simulink model "Quad"  (R2015a)
settings: Solver=ode3  StartTime=0.0  StopTime=10  FixedStep=0.01  RelTol=1e-3
settings Model: Creator=Nick  LastModifiedBy=Nick

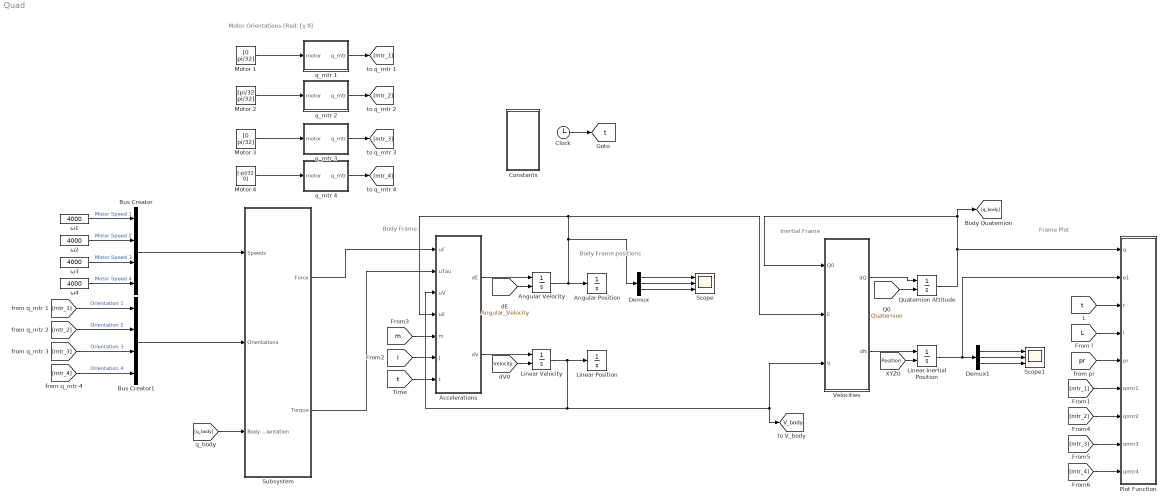
== system Quad ==
  note: Motor Orientations
      | (Rad: [γ δ]
  note: Frame Plot
  note: Inertial Frame
  note: Body Frame
      | positions
  note: Body Frame
  Accelerations : MATLAB Function  TreatAsAtomicUnit=on
  Angular Position : Integrator
  Angular Velocity : Integrator  InitialConditionSource=external
  Bus Creator : BusCreator
  Bus Creator1 : BusCreator
  Clock : Clock
  Constants : Subsystem
  Demux : Demux  Outputs=3
  Demux1 : Demux  Outputs=3
  Linear Inertial Position : Integrator  InitialConditionSource=external
  Linear Position : Integrator
  Linear Velocity : Integrator  InitialConditionSource=external
  Motor 1 : Constant  Value=[0 pi/32]
  Motor 2 : Constant  Value=[pi/32 pi/32]
  Motor 3 : Constant  Value=[0 pi/32]
  Motor 4 : Constant  Value=[-pi/32 0]
  Plot Function : MATLAB Function  TreatAsAtomicUnit=on
  Quaternion Attitude : Integrator  InitialConditionSource=external  ContinuousStateAttributes='Quaternion'
  Scope : Scope  NumInputPorts=3
      settings: YMin=-5~-5~-5  YMax=5~5~5
  Scope1 : Scope  NumInputPorts=3
      settings: YMin=-5~-5~-5  YMax=5~5~5
  Subsystem : Subsystem
  Velocities : MATLAB Function  TreatAsAtomicUnit=on
  q_mtr 1 : MATLAB Function  TreatAsAtomicUnit=on
  q_mtr 2 : MATLAB Function  TreatAsAtomicUnit=on
  q_mtr 3 : MATLAB Function  TreatAsAtomicUnit=on
  q_mtr 4 : MATLAB Function  TreatAsAtomicUnit=on
  ω{1..4} (4 alike) : Constant  Value=4000
  tag scope: V_body=global, t=global
  wires:
  [L] -> Plot Function/4(l)
  [pr] -> Plot Function/5(pr)
  Clock/1 -> [t]
  [t] -> Plot Function/3(t)
  [t] -> Accelerations/7(t)
  [I] -> Accelerations/6(J)
  [m] -> Accelerations/5(m)
  Accelerations/1(dE) -> Angular Velocity/1
  Angular Velocity/1 -> Demux/1, Accelerations/4(uE), Velocities/2(E), Angular Position/1
  Accelerations/2(dV) -> Linear Velocity/1
  Linear Velocity/1 -> Accelerations/3(uV), Velocities/3(V), [V_body], Linear Position/1
  Demux/1 -> Scope/1
  Demux/2 -> Scope/2
  Demux/3 -> Scope/3
  Demux1/1 -> Scope1/1
  Demux1/2 -> Scope1/2
  Demux1/3 -> Scope1/3
  [Velocity] -> Linear Velocity/2
  [Angular_Velocity] -> Angular Velocity/2
  Velocities/2(dN) -> Linear Inertial Position/1
  [Position] -> Linear Inertial Position/2
  Linear Inertial Position/1 -> Demux1/1, Plot Function/2(e1)
  [Quaternion] -> Quaternion Attitude/2
  Velocities/1(dQ) -> Quaternion Attitude/1
  Quaternion Attitude/1 -> [q_body], Velocities/1(Q0), Plot Function/1(q)
  Motor 1/1 -> q_mtr 1/1(motor)
  Motor 2/1 -> q_mtr 2/1(motor)
  Motor 3/1 -> q_mtr 3/1(motor)
  Motor 4/1 -> q_mtr 4/1(motor)
  q_mtr 1/1(q_mtr) -> [mtr_1]
  q_mtr 4/1(q_mtr) -> [mtr_4]
  q_mtr 3/1(q_mtr) -> [mtr_3]
  q_mtr 2/1(q_mtr) -> [mtr_2]
  [mtr_1] -> Plot Function/6(qmtr1)
  [mtr_2] -> Plot Function/7(qmtr2)
  [mtr_3] -> Plot Function/8(qmtr3)
  [mtr_4] -> Plot Function/9(qmtr4)
  [q_body] -> Subsystem/3(Body Orientation)
  Subsystem/1(Force) -> Accelerations/1(uF)
  Subsystem/2(Torque) -> Accelerations/2(uTau)
  ω1/1 -> Bus Creator/1  "Motor Speed 1"
  ω2/1 -> Bus Creator/2  "Motor Speed 2"
  ω3/1 -> Bus Creator/3  "Motor Speed 3"
  ω4/1 -> Bus Creator/4  "Motor Speed 4"
  Bus Creator/1 -> Subsystem/1(Speeds)
  [mtr_1] -> Bus Creator1/1  "Orientation 1"
  [mtr_2] -> Bus Creator1/2  "Orientation 2"
  [mtr_3] -> Bus Creator1/3  "Orientation 3"
  [mtr_4] -> Bus Creator1/4  "Orientation 4"
  Bus Creator1/1 -> Subsystem/2(Orientations)

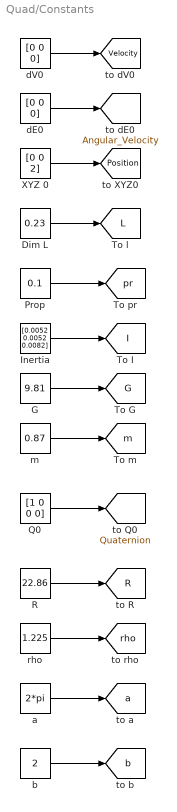
== system Quad/Constants ==
  Dim L : Constant  Value=0.23
  G : Constant  Value=9.81
  Inertia : Constant  Value=[0.0052 0.0052 0.0082]
  Prop : Constant  Value=0.1
  Q0 : Constant  Value=[1 0 0 0]
  R : Constant  Value=22.86
  XYZ 0 : Constant  Value=[0 0 2]
  a : Constant  Value=2*pi
  b : Constant  Value=2
  dE0 : Constant  Value=[0 0 0]
  dV0 : Constant  Value=[0 0 0]
  m : Constant  Value=0.87
  rho : Constant  Value=1.225
  tag scope: Angular_Velocity=global, G=global, I=global, L=global, Position=global, Quaternion=global, R=global, Velocity=global, a=global, b=global, m=global, pr=global, rho=global
  wires:
  XYZ 0/1 -> [Position]
  Dim L/1 -> [L]
  Prop/1 -> [pr]
  Inertia/1 -> [I]
  G/1 -> [G]
  m/1 -> [m]
  dV0/1 -> [Velocity]
  dE0/1 -> [Angular_Velocity]
  Q0/1 -> [Quaternion]
  R/1 -> [R]
  rho/1 -> [rho]
  a/1 -> [a]
  b/1 -> [b]

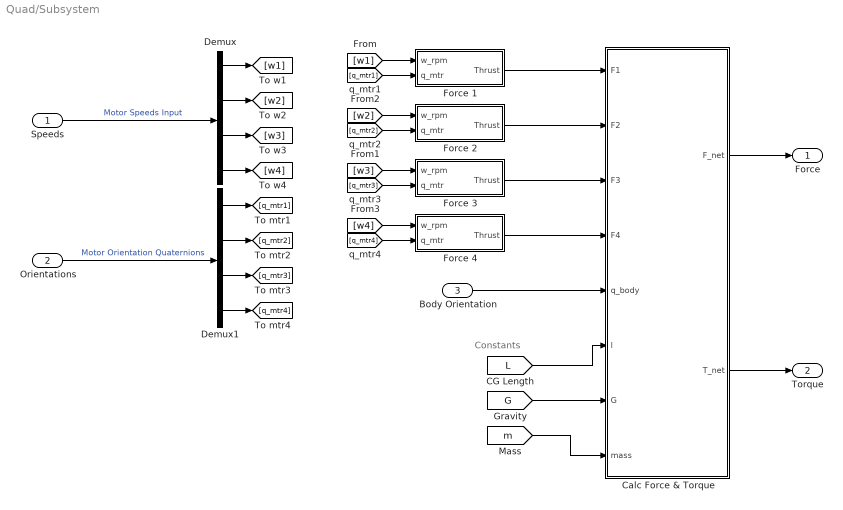
== system Quad/Subsystem ==
  note: Constants
  Speeds : Inport  PortDimensions=4
  Orientations : Inport  Port=2  PortDimensions=16
  Body Orientation : Inport  Port=3
  Calc Force & Torque : MATLAB Function  TreatAsAtomicUnit=on
  Demux : Demux
  Demux1 : Demux
  Force 1 : Subsystem
  Force 2 : Subsystem
  Force 3 : Subsystem
  Force 4 : Subsystem
  Force : Outport
  Torque : Outport  Port=2
  wires:
  Calc Force & Torque/1(F_net) -> Force/1
  [L] -> Calc Force & Torque/6(l)
  Body Orientation/1 -> Calc Force & Torque/5(q_body)
  [m] -> Calc Force & Torque/8(mass)
  Speeds/1 -> Demux/1  "Motor Speeds Input"
  Orientations/1 -> Demux1/1  "Motor Orientation Quaternions"
  Calc Force & Torque/2(T_net) -> Torque/1
  [G] -> Calc Force & Torque/7(G)
  Demux/1 -> [w1]
  Demux/2 -> [w2]
  Demux/3 -> [w3]
  Demux/4 -> [w4]
  Demux1/1 -> [q_mtr1]
  Demux1/2 -> [q_mtr2]
  Demux1/3 -> [q_mtr3]
  Demux1/4 -> [q_mtr4]
  [w1] -> Force 1/1(w_rpm)
  [q_mtr1] -> Force 1/2(q_mtr)
  Force 1/1(Thrust) -> Calc Force & Torque/1(F1)
  Force 2/1(Thrust) -> Calc Force & Torque/2(F2)
  [w2] -> Force 2/1(w_rpm)
  [q_mtr2] -> Force 2/2(q_mtr)
  Force 3/1(Thrust) -> Calc Force & Torque/3(F3)
  [w3] -> Force 3/1(w_rpm)
  [q_mtr3] -> Force 3/2(q_mtr)
  Force 4/1(Thrust) -> Calc Force & Torque/4(F4)
  [w4] -> Force 4/1(w_rpm)
  [q_mtr4] -> Force 4/2(q_mtr)

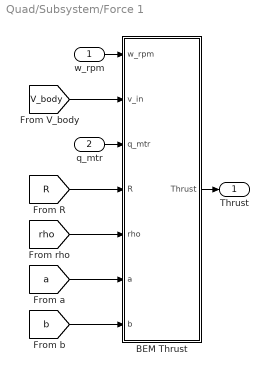
== system Quad/Subsystem/Force 1 ==
  w_rpm : Inport
  q_mtr : Inport  Port=2
  BEM Thrust : MATLAB Function  TreatAsAtomicUnit=on
  Thrust : Outport
  wires:
  [a] -> BEM Thrust/6(a)
  [b] -> BEM Thrust/7(b)
  [V_body] -> BEM Thrust/2(v_in)
  [rho] -> BEM Thrust/5(rho)
  [R] -> BEM Thrust/4(R)
  q_mtr/1 -> BEM Thrust/3(q_mtr)
  BEM Thrust/1(Thrust) -> Thrust/1
  w_rpm/1 -> BEM Thrust/1(w_rpm)

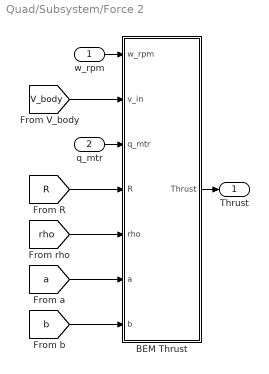
== system Quad/Subsystem/Force 2 ==
  w_rpm : Inport
  q_mtr : Inport  Port=2
  BEM Thrust : MATLAB Function  TreatAsAtomicUnit=on
  Thrust : Outport
  wires:
  [a] -> BEM Thrust/6(a)
  [b] -> BEM Thrust/7(b)
  [V_body] -> BEM Thrust/2(v_in)
  [rho] -> BEM Thrust/5(rho)
  [R] -> BEM Thrust/4(R)
  q_mtr/1 -> BEM Thrust/3(q_mtr)
  BEM Thrust/1(Thrust) -> Thrust/1
  w_rpm/1 -> BEM Thrust/1(w_rpm)

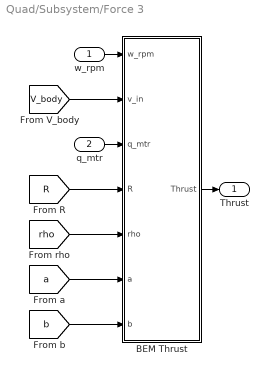
== system Quad/Subsystem/Force 3 ==
  w_rpm : Inport
  q_mtr : Inport  Port=2
  BEM Thrust : MATLAB Function  TreatAsAtomicUnit=on
  Thrust : Outport
  wires:
  [a] -> BEM Thrust/6(a)
  [b] -> BEM Thrust/7(b)
  [V_body] -> BEM Thrust/2(v_in)
  [rho] -> BEM Thrust/5(rho)
  [R] -> BEM Thrust/4(R)
  q_mtr/1 -> BEM Thrust/3(q_mtr)
  BEM Thrust/1(Thrust) -> Thrust/1
  w_rpm/1 -> BEM Thrust/1(w_rpm)

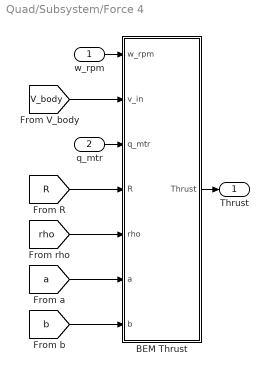
== system Quad/Subsystem/Force 4 ==
  w_rpm : Inport
  q_mtr : Inport  Port=2
  BEM Thrust : MATLAB Function  TreatAsAtomicUnit=on
  Thrust : Outport
  wires:
  [a] -> BEM Thrust/6(a)
  [b] -> BEM Thrust/7(b)
  [V_body] -> BEM Thrust/2(v_in)
  [rho] -> BEM Thrust/5(rho)
  [R] -> BEM Thrust/4(R)
  q_mtr/1 -> BEM Thrust/3(q_mtr)
  BEM Thrust/1(Thrust) -> Thrust/1
  w_rpm/1 -> BEM Thrust/1(w_rpm)

== matlab function Quad/Subsystem/Calc Force & Torque ==
  data: F_net output; F1 input; F2 input; F3 input; F4 input; q_body input; T_net output size=1 3; l input; G input; mass input
function [F_net,T_net] = motor_dynamics(F1,F2,F3,F4,q_body,l,G,mass)
%%Gravity Vector -> Inertial Frame
F_g_w = [0 0 0 -mass*G];
%%Body Frame Quaternion
Q_b = quatnormalize([q_body(1) q_body(2) q_body(3) q_body(4)]);
Q_b_conj = quatconj(Q_b);
%%Motor Forces -> Body Frame
q_F1 = [0 F1(1) F1(2) F1(3)];
q_F2 = [0 F2(1) F2(2) F2(3)];
q_F3 = [0 F3(1) F3(2) F3(3)];
q_F4 = [0 F4(1) F4(2) F4(3)];
%%Net Motor Forces -> Body Frame
q_F_m = q_F1 + q_F2 + q_F3 + q_F4; 
%%Gravity Vector -> Body Frame
F_g_b = quatmultiply((quatmultiply(Q_b,F_g_w)),Q_b_conj);
%%F_net summed together 
q_F = q_F_m + F_g_b; % + D
F_net = [q_F(2) q_F(3) q_F(4)];
%%Differential Torques -> Body Frame
T_diff_x = l*q_F1(4) - l*q_F3(4);
T_diff_y = l*q_F2(4) - l*q_F4(4);
T_diff_z = l*q_F1(2) - l*q_F3(2) + l*q_F2(1) - l*q_F4(1);
T_diff = [T_diff_x T_diff_y T_diff_z];
%%T_net Summed together
T = T_diff; % + G + M
T_net = [T(1) T(2) T(3)];
%disp(T_net);
%disp(F_net);
end

== matlab function Quad/Accelerations ==
  data: uF input; uTau input; uV input; uE input; m input; J input; t input; dE output; dV output
function [dE,dV]= Dynamics(uF,uTau,uV,uE,m,J,t) %#ok<*INUSD>
mass = m; %variable mass
%%Mass Moment of Inertia
J_x = J(1);
J_y = J(2);
J_z = J(3); %Kg.Nm
%%control action
%%All in F_b
%%Force Inputs
f_x = uF(1);
f_y = uF(2);
f_z = uF(3);
F = [f_x f_y f_z]; %N
%%Torque Inputs
t_phi = uTau(1);
t_theta = uTau(2);
t_rho = uTau(3);
Tau = [t_phi t_theta t_rho]; %Nm
%%current state translational velocity
u = uV(1);
v = uV(2);
w = uV(3);
V = [u v w]; %m.s^-1
%%current state angular velocity
p = uE(1);
q = uE(2);
r = uE(3);
E = [p q r]; %rad.s^-1
%%Angular accelerations in Body Frame
dp = (1/J_x)*((J_y-J_z)*q*r+t_phi);
dq = (1/J_y)*((J_z-J_x)*p*r+t_theta);
dr = (1/J_z)*((J_x-J_y)*p*q+t_rho);
dE = zeros(3,1); %rad.s^-2
dE(1)=dp;
dE(2)=dq;
dE(3)=dr;
%%Linear accelerations in Body Frame
dV = cross(E,V)+(1/mass)*F; %m.s^-2
%Integrals take place outside dynamics function
end

== matlab function Quad/Plot Function ==
  data: q input; e1 input; t input; l input; pr input; qmtr1 input; qmtr2 input; qmtr3 input; qmtr4 input
function plot(q,e1,t,l,pr,qmtr1,qmtr2,qmtr3,qmtr4)
%Input t
%CG Cartesian Co-ordinates
X = e1(1); %X Position
Y = e1(2); %Y Position
Z = e1(3); %Z Position
%Calculate Motor Positions relative to 0;0;0
%l may be variable
XYmtr1 = ([l 0 0]);
XYmtr2 = ([0 l 0]);
XYmtr3 = ([-l 0 0]);
XYmtr4 = ([0 -l 0]);
%%Calculate Body Attidue (Normal Vector)
Q = quatnormalize(q.'); %Body Quaternion, read from d/dt(Q)
Q_conj = quatconj(Q);   %Quaternion conjugate
N_b = [0 0 1];      %normal vector in Body frame
L_b = [0 N_b(1) N_b(2) N_b(3)]; %Build normal quaternion
L1 = quatmultiply(Q_conj,L_b);
L2 = quatmultiply(L1,Q);    %Normal rotated by Body Quaternion
N_w = [L2(2) L2(3) L2(4)];  %Normal vector in inertial frame
%%Calculate Motor 1 Attitudes
Q_XYmtr1 = [0 XYmtr1(1) XYmtr1(2) XYmtr1(3)]; %XYZ position of motor 1 from CG
L1 = quatmultiply(Q_conj,Q_XYmtr1);
L2 = quatmultiply(L1,Q);    %Rotate rotor arm by body quaternion
mtr1_w = e1.' + [L2(2) L2(3) L2(4)]; %Calculate new XYZ position using attitude quaternion
L_1 = [0 0 0 1];       %k considered to be normal for motor 1 (Force acting just in the Z-direction)
Q_mtr1 = [qmtr1(1) qmtr1(2) qmtr1(3) qmtr1(4)]; %Calculate motor 1 attitude from motor 1 quaternion
Q_mtr1_conj = quatconj(Q_mtr1);
L1 = quatmultiply(Q_mtr1_conj,L_1);
L2 = quatmultiply(L1,Q_mtr1);
L3 = quatmultiply(Q_conj,L2);
L4 = quatmultiply(L3,Q);
mtr1_N = [L4(2) L4(3) L4(4)]; %Motor 1 Normal Vector
%%Calculate Motor 3 Attitudes
Q_XYmtr3 = [0 XYmtr3(1) XYmtr3(2) XYmtr3(3)];
L1 = quatmultiply(Q_conj,Q_XYmtr3);
L2 = quatmultiply(L1,Q);
mtr3_w = e1.' + [L2(2) L2(3) L2(4)];
L_3 = [0 0 0 1];
Q_mtr3 = [qmtr3(1) qmtr3(2) qmtr3(3) qmtr3(4)]; %Calculate motor 3 attitude from motor 3 quaternion
Q_mtr3_conj = quatconj(Q_mtr3);
L1 = quatmultiply(Q_mtr3_conj,L_3);
L2 = quatmultiply(L1,Q_mtr3);
L3 = quatmultiply(Q_conj,L2);
L4 = quatmultiply(L3,Q);
mtr3_N = [L4(2) L4(3) L4(4)]; %Motor 3 Normal Vector
%%Calculate Motor 2 Attitudes
Q_XYmtr2 = [0 XYmtr2(1) XYmtr2(2) XYmtr2(3)];
L1 = quatmultiply(Q_conj,Q_XYmtr2);
L2 = quatmultiply(L1,Q);
mtr2_w = e1.' + [L2(2) L2(3) L2(4)];
L_2 = [0 0 0 1];
Q_mtr2 = [qmtr2(1) qmtr2(2) qmtr2(3) qmtr2(4)]; %Calculate motor 2 attitude from motor 2 quaternion
Q_mtr2_conj = quatconj(Q_mtr2);
L1 = quatmultiply(Q_mtr2_conj,L_2);
L2 = quatmultiply(L1,Q_mtr2);
L3 = quatmultiply(Q_conj,L2);
L4 = quatmultiply(L3,Q);
mtr2_N = [L4(2) L4(3) L4(4)]; %Motor 2 Normal Vector
%%Calculate Motor 4 Attitudes
Q_XYmtr4 = [0 XYmtr4(1) XYmtr4(2) XYmtr4(3)];
L1 = quatmultiply(Q_conj,Q_XYmtr4);
L2 = quatmultiply(L1,Q);
mtr4_w = e1.' + [L2(2) L2(3) L2(4)];
L_4 = [0 0 0 1];
Q_mtr4 = [qmtr4(1) qmtr4(2) qmtr4(3) qmtr4(4)]; %Calculate motor 2 attitude from motor 2 quaternion
Q_mtr4_conj = quatconj(Q_mtr4);
L1 = quatmultiply(Q_mtr4_conj,L_4);
L2 = quatmultiply(L1,Q_mtr4);
L3 = quatmultiply(Q_conj,L2);
L4 = quatmultiply(L3,Q);
mtr4_N = [L4(2) L4(3) L4(4)]; %Motor 2 Normal Vector
%%Open Figure if first time instance
if(t==0);
    fig = figure();
    hold on;
    grid on;
end
%%Clear and Construct Figure
hold off;
clf();
xlim([-1 5]);
ylim([-1 5]);
zlim([0 5]);
view([4 4 5]);
grid on;
hold on;
%%Display Time
%disp(t);
%%Plot Quad Function
plotCircle3D([X Y 0],[0 0 1],(l),'black');
plot3(([mtr1_w(1) mtr3_w(1)]),([mtr1_w(2) mtr3_w(2)]),([mtr1_w(3) mtr3_w(3)]),'LineWidth',1,'Color','Blue');
plot3(([mtr2_w(1) mtr4_w(1)]),([mtr2_w(2) mtr4_w(2)]),([mtr2_w(3) mtr4_w(3)]),'LineWidth',1,'Color','Blue');
plotCircle3D(mtr1_w,mtr1_N,pr,'red');
plotCircle3D(mtr2_w,mtr2_N,pr,'red');
plotCircle3D(mtr3_w,mtr3_N,pr,'red');
plotCircle3D(mtr4_w,mtr4_N,pr,'red');
plotCircle3D([X Y Z],N_w,(l+pr),'green');
%%
end

== matlab function Quad/Subsystem/Force 1/BEM Thrust ==
  data: w_rpm input; Thrust output; v_in input; q_mtr input; R input; rho input; a input; b input
function Thrust = fthrust(w_rpm,v_in,q_mtr,R,rho,a,b)
w_rads = (w_rpm/60)*2*pi; %rad.s^-1
%v_inf incident velocity ms^-1
%R propeller radius cm
%rho kg.m^3
%a lift curve slope
%b rotors
Q = [q_mtr(1) q_mtr(2) q_mtr(3) q_mtr(4)]; %quaternion motor orientation
Q = quatnormalize(Q);
Q_conj = quatconj(Q); %quaternion conjugate
v_in_b = [0 v_in(1) v_in(2) v_in(3)]; %vehicle velocity in body frame
v_in_m = quatmultiply(Q,(quatmultiply(v_in_b,Q_conj))); %vehicle velocity in motor frame
v_inf = v_in_m(4); %perpendicular Z component of vehicle velocity
T = 0; %initialize thrust
for r = 0.15*R:0.01:R %integrate 0.15R -> R
    x = r/R; %ratio of r to R
    Cr_R = ((5623*x^6)/1000 - (2221*x^5)/100 + (173*x^4)/5 - (683*x^3)/25 + (1079*x^2)/100 - (813*x)/500 + 1987/10000)*(10^-3); %chord length (m*10^-2)
    Br_R = - (731*x^6)/20 + 138*x^5 - 210*x^4 + (1637*x^3)/10 - (3383*x^2)/50 + (643*x)/50 - 2003/10000; %local angle of attack rad
    gamma_c = (v_inf)./(w_rads.*(R*10^-3)); %static inflow factor
    sigma = (b*Cr_R)/(pi*R*10^-3); %blade solidity
    gamma = sqrt((sigma*a/16 - gamma_c/2).^2 + (sigma*a/8)*Br_R*x)-(sigma*a/16 - gamma_c/2); %inflow factor
    dT = a*b*Cr_R*(rho/2)*(w_rads.*r*10^-3).^2.*(Br_R - gamma); %thrust element
    T = T + dT; %calculate integral
end
disp(T);
T_q = [0 0 0 T/10]; %quaternion thrust vector in motor frame
T_q_b = quatmultiply(Q_conj,quatmultiply(T_q,Q)); %thrust quaternion in body frame
Thrust = [T_q_b(2) T_q_b(3) T_q_b(4)]; %thrust vector in body frame
end

== matlab function Quad/Velocities ==
  data: Q0 input; dQ output; E input; V input; dN output
function [dQ,dN] = inertialdynamics(Q0,E,V)
%#codegen
V1 = V.';
qE = [0 E(1) E(2) E(3)];
Q = quatnormalize(Q0.');
Q_conj = quatconj(Q);
dQ=(1/2)*quatmultiply(Q,qE);
%ndQ = quatnormalize(dQ);
V2 = [0 V1(1) V1(2) V1(3)];
L1 = quatmultiply(Q_conj,V2);
L2 = quatmultiply(L1,Q);
dN = [L2(2) L2(3) L2(4)];
end

== matlab function Quad/q_mtr 1 ==
  data: motor input; q_mtr output
function q_mtr = quat_convert(motor)
q_mtr = zeros(1,4);
gamma = motor(1);
delta = motor(2);
q_gamma = [cos(gamma/2) 0 sin(gamma/2) 0];
q_delta = [cos(delta/2) sin(delta/2) 0 0];
q = quatmultiply(q_gamma,q_delta);
q_mtr = quatnormalize(q);
end

== matlab function Quad/q_mtr 2 ==
  data: motor input; q_mtr output
function q_mtr = quat_convert(motor)
q_mtr = zeros(1,4);
gamma = motor(1);
delta = motor(2);
q_gamma = [cos(gamma/2) 0 sin(gamma/2) 0];
q_delta = [cos(delta/2) sin(delta/2) 0 0];
q = quatmultiply(q_gamma,q_delta);
q_mtr = quatnormalize(q);
end

== matlab function Quad/q_mtr 3 ==
  data: motor input; q_mtr output
function q_mtr = quat_convert(motor)
q_mtr = zeros(1,4);
gamma = motor(1);
delta = motor(2);
q_gamma = [cos(gamma/2) 0 sin(gamma/2) 0];
q_delta = [cos(delta/2) sin(delta/2) 0 0];
q = quatmultiply(q_gamma,q_delta);
q_mtr = quatnormalize(q);
end

== matlab function Quad/q_mtr 4 ==
  data: motor input; q_mtr output
function q_mtr = quat_convert(motor)
q_mtr = zeros(1,4);
gamma = motor(1);
delta = motor(2);
q_gamma = [cos(gamma/2) 0 sin(gamma/2) 0];
q_delta = [cos(delta/2) sin(delta/2) 0 0];
q = quatmultiply(q_gamma,q_delta);
q_mtr = quatnormalize(q);
end

== matlab function Quad/Subsystem/Force 2/BEM Thrust ==
  data: w_rpm input; Thrust output; v_in input; q_mtr input; R input; rho input; a input; b input
function Thrust = fthrust(w_rpm,v_in,q_mtr,R,rho,a,b)
w_rads = (w_rpm/60)*2*pi; %rad.s^-1
%v_inf incident velocity ms^-1
%R propeller radius cm
%rho kg.m^3
%a lift curve slope
%b rotors
Q = [q_mtr(1) q_mtr(2) q_mtr(3) q_mtr(4)]; %quaternion motor orientation
Q = quatnormalize(Q);
Q_conj = quatconj(Q); %quaternion conjugate
v_in_b = [0 v_in(1) v_in(2) v_in(3)]; %vehicle velocity in body frame
v_in_m = quatmultiply(Q,(quatmultiply(v_in_b,Q_conj))); %vehicle velocity in motor frame
v_inf = v_in_m(4); %perpendicular Z component of vehicle velocity
T = 0; %initialize thrust
for r = 0.15*R:0.01:R %integrate 0.15R -> R
    x = r/R; %ratio of r to R
    Cr_R = ((5623*x^6)/1000 - (2221*x^5)/100 + (173*x^4)/5 - (683*x^3)/25 + (1079*x^2)/100 - (813*x)/500 + 1987/10000)*(10^-3); %chord length (m*10^-2)
    Br_R = - (731*x^6)/20 + 138*x^5 - 210*x^4 + (1637*x^3)/10 - (3383*x^2)/50 + (643*x)/50 - 2003/10000; %local angle of attack rad
    gamma_c = (v_inf)./(w_rads.*(R*10^-3)); %static inflow factor
    sigma = (b*Cr_R)/(pi*R*10^-3); %blade solidity
    gamma = sqrt((sigma*a/16 - gamma_c/2).^2 + (sigma*a/8)*Br_R*x)-(sigma*a/16 - gamma_c/2); %inflow factor
    dT = a*b*Cr_R*(rho/2)*(w_rads.*r*10^-3).^2.*(Br_R - gamma); %thrust element
    T = T + dT; %calculate integral
end
disp(T);
T_q = [0 0 0 T/10]; %quaternion thrust vector in motor frame
T_q_b = quatmultiply(Q_conj,quatmultiply(T_q,Q)); %thrust quaternion in body frame
Thrust = [T_q_b(2) T_q_b(3) T_q_b(4)]; %thrust vector in body frame
end

== matlab function Quad/Subsystem/Force 3/BEM Thrust ==
  data: w_rpm input; Thrust output; v_in input; q_mtr input; R input; rho input; a input; b input
function Thrust = fthrust(w_rpm,v_in,q_mtr,R,rho,a,b)
w_rads = (w_rpm/60)*2*pi; %rad.s^-1
%v_inf incident velocity ms^-1
%R propeller radius cm
%rho kg.m^3
%a lift curve slope
%b rotors
Q = [q_mtr(1) q_mtr(2) q_mtr(3) q_mtr(4)]; %quaternion motor orientation
Q = quatnormalize(Q);
Q_conj = quatconj(Q); %quaternion conjugate
v_in_b = [0 v_in(1) v_in(2) v_in(3)]; %vehicle velocity in body frame
v_in_m = quatmultiply(Q,(quatmultiply(v_in_b,Q_conj))); %vehicle velocity in motor frame
v_inf = v_in_m(4); %perpendicular Z component of vehicle velocity
T = 0; %initialize thrust
for r = 0.15*R:0.01:R %integrate 0.15R -> R
    x = r/R; %ratio of r to R
    Cr_R = ((5623*x^6)/1000 - (2221*x^5)/100 + (173*x^4)/5 - (683*x^3)/25 + (1079*x^2)/100 - (813*x)/500 + 1987/10000)*(10^-3); %chord length (m*10^-2)
    Br_R = - (731*x^6)/20 + 138*x^5 - 210*x^4 + (1637*x^3)/10 - (3383*x^2)/50 + (643*x)/50 - 2003/10000; %local angle of attack rad
    gamma_c = (v_inf)./(w_rads.*(R*10^-3)); %static inflow factor
    sigma = (b*Cr_R)/(pi*R*10^-3); %blade solidity
    gamma = sqrt((sigma*a/16 - gamma_c/2).^2 + (sigma*a/8)*Br_R*x)-(sigma*a/16 - gamma_c/2); %inflow factor
    dT = a*b*Cr_R*(rho/2)*(w_rads.*r*10^-3).^2.*(Br_R - gamma); %thrust element
    T = T + dT; %calculate integral
end
disp(T);
T_q = [0 0 0 T/10]; %quaternion thrust vector in motor frame
T_q_b = quatmultiply(Q_conj,quatmultiply(T_q,Q)); %thrust quaternion in body frame
Thrust = [T_q_b(2) T_q_b(3) T_q_b(4)]; %thrust vector in body frame
end

== matlab function Quad/Subsystem/Force 4/BEM Thrust ==
  data: w_rpm input; Thrust output; v_in input; q_mtr input; R input; rho input; a input; b input
function Thrust = fthrust(w_rpm,v_in,q_mtr,R,rho,a,b)
w_rads = (w_rpm/60)*2*pi; %rad.s^-1
%v_inf incident velocity ms^-1
%R propeller radius cm
%rho kg.m^3
%a lift curve slope
%b rotors
Q = [q_mtr(1) q_mtr(2) q_mtr(3) q_mtr(4)]; %quaternion motor orientation
Q = quatnormalize(Q);
Q_conj = quatconj(Q); %quaternion conjugate
v_in_b = [0 v_in(1) v_in(2) v_in(3)]; %vehicle velocity in body frame
v_in_m = quatmultiply(Q,(quatmultiply(v_in_b,Q_conj))); %vehicle velocity in motor frame
v_inf = v_in_m(4); %perpendicular Z component of vehicle velocity
T = 0; %initialize thrust
for r = 0.15*R:0.01:R %integrate 0.15R -> R
    x = r/R; %ratio of r to R
    Cr_R = ((5623*x^6)/1000 - (2221*x^5)/100 + (173*x^4)/5 - (683*x^3)/25 + (1079*x^2)/100 - (813*x)/500 + 1987/10000)*(10^-3); %chord length (m*10^-2)
    Br_R = - (731*x^6)/20 + 138*x^5 - 210*x^4 + (1637*x^3)/10 - (3383*x^2)/50 + (643*x)/50 - 2003/10000; %local angle of attack rad
    gamma_c = (v_inf)./(w_rads.*(R*10^-3)); %static inflow factor
    sigma = (b*Cr_R)/(pi*R*10^-3); %blade solidity
    gamma = sqrt((sigma*a/16 - gamma_c/2).^2 + (sigma*a/8)*Br_R*x)-(sigma*a/16 - gamma_c/2); %inflow factor
    dT = a*b*Cr_R*(rho/2)*(w_rads.*r*10^-3).^2.*(Br_R - gamma); %thrust element
    T = T + dT; %calculate integral
end
disp(T);
T_q = [0 0 0 T/10]; %quaternion thrust vector in motor frame
T_q_b = quatmultiply(Q_conj,quatmultiply(T_q,Q)); %thrust quaternion in body frame
Thrust = [T_q_b(2) T_q_b(3) T_q_b(4)]; %thrust vector in body frame
end
